simulink model "h2aps_version_final"  (R2024b)
settings: Solver=VariableStepAuto  StartTime=0.0  StopTime=10  RelTol=1e-3
InitFcn:
  | Ts = 1000e-6;
StartFcn:
  | Ts = 1000e-6;
undefined symbols (not defined in the file or in its folder): Ion, Lithium
libraries: slpidlib x13, spsCurrentMeasurementLib x13, simulink x11, spsVoltageMeasurementLib x10, spsSeriesRLCBranchLib x8, spsIGBTDiodeLib x5, spspowerguiLib x2, spsDiodeLib x2, spsBatteryLib x1, spsDCVoltageSourceLib x1, spsVariableResistorLib x1, spsIGBTLib x1
(part 2 of 2)

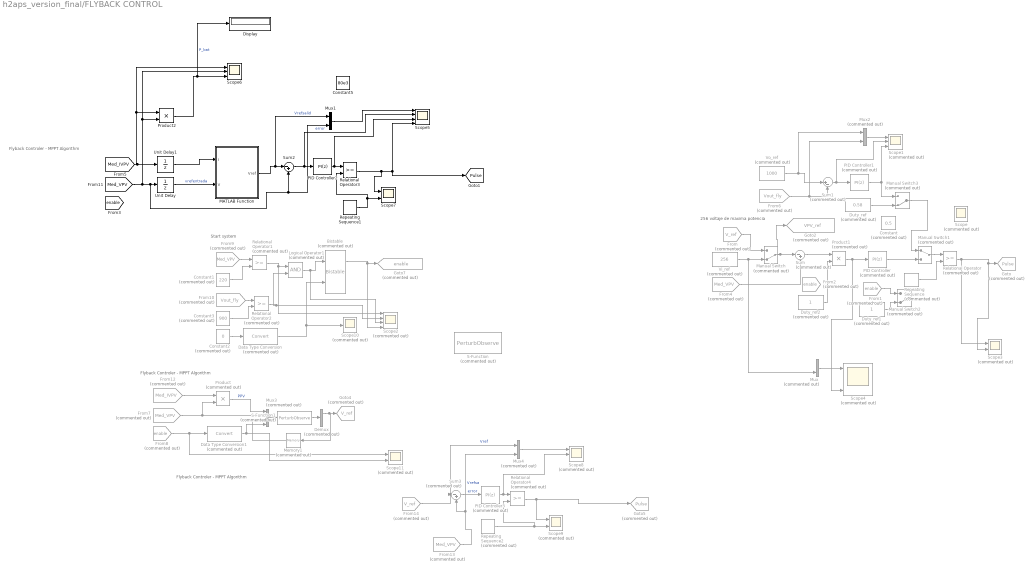
== system h2aps_version_final/FLYBACK CONTROL ==
  note: 256 voltaje de maxima potencia
  note: Flyback Controler - MPPT Algorithm
  note: Start system
  note: Flyback Controler - MPPT Algorithm
  note: Flyback Controler - MPPT Algorithm
  Bistable : spsBistableLib/Bistable  Commented=on  Qpriority=Set  ic=0  Ts=0
      settings: LibrarySourceBlock=sps_lib/Control/Bistable
  Constant : Constant  Commented=on  Value=0.5
  Constant1 : Constant  Commented=on  Value=220
  Constant2 : Constant  Commented=on  Value=0
  Constant3 : Constant  Commented=on  Value=900
  Constant5 : Constant  Value=80e3
  Data Type Conversion : DataTypeConversion  Commented=on  SaturateOnIntegerOverflow=off  RndMeth=Floor
  Data Type Conversion1 : DataTypeConversion  Commented=on  SaturateOnIntegerOverflow=off  RndMeth=Floor
  Demux : Demux  Commented=on  Outputs=3
  Display : Display
  Duty_ref : Constant  Commented=on  Value=0.58
  Duty_ref1 : Constant  Commented=on
  Duty_ref2 : Constant  Commented=on
  From : From  Commented=on  GotoTag=V_ref
  From1 : From  Commented=on  GotoTag=enable
  From10 : From  Commented=on  GotoTag=Vout_fly  TagVisibility=global
  From12 : From  Commented=on  GotoTag=Med_IVPV  TagVisibility=global
  From{4,7,9,13} (4 alike) : From  Commented=on  GotoTag=Med_VPV  TagVisibility=global
  From14 : From  Commented=on  GotoTag=V_ref  TagVisibility=global
  From2 : From  Commented=on  GotoTag=enable
  From6 : From  Commented=on  GotoTag=Vout_fly  TagVisibility=global
  From8 : From  Commented=on  GotoTag=enable  TagVisibility=global
  Goto : Goto  Commented=on  GotoTag=Pulse  TagVisibility=global
  Goto2 : Goto  Commented=on  GotoTag=VPV_ref  TagVisibility=global
  Goto4 : Goto  Commented=on  GotoTag=V_ref  TagVisibility=global
  Goto5 : Goto  Commented=on  GotoTag=Pulse  TagVisibility=global
  Goto7 : Goto  Commented=on  GotoTag=enable  TagVisibility=global
  Logical Operator1 : Logic  Commented=on  AllPortsSameDT=off  OutDataTypeStr=boolean
  MATLAB Function : MATLAB Function  TreatAsAtomicUnit=on
  Manual Switch : ManualSwitch  Commented=on  CurrentSetting=0
  Manual Switch1 : ManualSwitch  Commented=on
  Manual Switch2 : ManualSwitch  Commented=on  CurrentSetting=0
  Manual Switch3 : ManualSwitch  Commented=on  CurrentSetting=0
  Memory1 : Memory  Commented=on
  Mux : Mux  Commented=on  Inputs=2
  Mux1 : Mux  Inputs=2
  Mux2 : Mux  Commented=on  Inputs=2
  Mux3 : Mux  Commented=on
  Mux4 : Mux  Commented=on  Inputs=2
  PID Controller : slpidlib/PID Controller  Commented=on  Controller=PI  Form=Parallel  TimeDomain=Discrete-time  UseExternalTs=off  SampleTime=Ts  IntegratorMethod=Forward Euler  FilterMethod=Forward Euler  ControllerParametersSource=internal  P=0.02/3.2  I=0.04/(2.2*100e-3)  UseKiTs=off  D=0  UseExternalDerivativeSource=off  N=100  UseFilter=on  TunerSelectOption=Transfer Function Based (PID Tuner App)  InitialConditionSource=internal  InitialConditionForIntegrator=0  InitialConditionForFilter=0  DifferentiatorICPrevScaledInput=0  ExternalReset=none  TrackingMode=off  Kt=1  LimitOutput=on  SatLimitsSource=internal  UpperSaturationLimit=1  LowerSaturationLimit=0  LinearizeAsGain=on  AntiWindupMode=clamping  Kb=1  LimitIntegrator=off  UpperIntegratorSaturationLimit=inf  LowerIntegratorSaturationLimit=-inf  POutMin=[]  POutMax=[]  IOutMin=[]  IOutMax=[]  DOutMin=[]  DOutMax=[]  NOutMin=[]  NOutMax=[]  SumOutMin=[]  SumOutMax=[]  SaturationOutMin=[]  SaturationOutMax=[]  PParamMin=[]  PParamMax=[]  IParamMin=[]  IParamMax=[]  DParamMin=[]  DParamMax=[]  NParamMin=[]  NParamMax=[]  KbParamMin=[]  KbParamMax=[]  KtParamMin=[]  KtParamMax=[]  KbOutMin=[]  KbOutMax=[]  KtOutMin=[]  KtOutMax=[]  IntegratorOutMin=[]  IntegratorOutMax=[]  FilterOutMin=[]  FilterOutMax=[]  SumI1OutMin=[]  SumI1OutMax=[]  SumI2OutMin=[]  SumI2OutMax=[]  SumI3OutMin=[]  SumI3OutMax=[]  SumI4OutMin=[]  SumI4OutMax=[]  SumDOutMin=[]  SumDOutMax=[]  DifferentiatorOutMin=[]  DifferentiatorOutMax=[]  FilterDiffOutCoefMin=[]  FilterDiffOutCoefMax=[]  ReciprocalOutMin=[]  ReciprocalOutMax=[]  SumDenOutMin=[]  SumDenOutMax=[]  SumNumOutMin=[]  SumNumOutMax=[]  DivideOutMin=[]  DivideOutMax=[]  UdiffTsProdOutMin=[]  UdiffTsProdOutMax=[]  NTsProdOutMin=[]  NTsProdOutMax=[]  UintegralTsProdOutMin=[]  UintegralTsProdOutMax=[]  UngainTsProdOutMin=[]  UngainTsProdOutMax=[]  ClampingZeroOutDataTypeStr=Inherit: Inherit via back propagation  ClampingZeroOutMin=[]  ClampingZeroOutMax=[]  FilterDenConstantOutDataTypeStr=Inherit: Inherit via back propagation  FilterDenConstantOutMin=[]  FilterDenConstantOutMax=[]  PCopyOutDataTypeStr=Inherit: Inherit via back propagation  PCopyOutMin=[]  PCopyOutMax=[]  NCopyOutDataTypeStr=Inherit: Inherit via back propagation  NCopyOutMin=[]  NCopyOutMax=[]  IntegratorContinuousStateAttributes=''  IntegratorStateMustResolveToSignalObject=off  IntegratorRTWStateStorageClass=Auto  FilterContinuousStateAttributes=''  FilterStateMustResolveToSignalObject=off  FilterRTWStateStorageClass=Auto  ParallelPVariant=InternalParameters  IdealPVariant=Disabled  IVariant=InternalParameters  DVariant=Disabled  IntegratorVariant=Discrete  SatVariant=Enabled  AWVariant=DiscClampingParallel  PCopyVariant=Disabled  TRVariant=Disabled  FdbkBlocksVariant=Forward  IdealPFdbkVariant=Disabled  SatFdbkVariant=Disabled  DerivativeFilterVariant=Disabled  NVariant=Disabled  NCopyVariant=Disabled_SignalSpec  FilterICVariant=Disabled  IntegratorICVariant=InternalICs  ExternalResetVariant=Disabled  TRSumVariant=Passthrough  SumFdbkVariant=Disabled  SumVariant=Sum_PI  TsampFilterVariant=InternalTs  TsampNgainVariant=Passthrough  TsampIntegralVariant=Disabled_SignalSpec  ExternalSaturationOutDataTypeStr=Inherit: Same as second input  DerivativeSourceVariant=Disabled  PreIntVariant=InternalPreInt
  PID Controller1 : slpidlib/PID Controller  Commented=on  Controller=PI  Form=Parallel  TimeDomain=Discrete-time  UseExternalTs=off  SampleTime=Ts  IntegratorMethod=Forward Euler  FilterMethod=Forward Euler  ControllerParametersSource=internal  P=0.02/3.2  I=0.04/(2.2*100e-3)  UseKiTs=off  D=0  UseExternalDerivativeSource=off  N=100  UseFilter=on  TunerSelectOption=Transfer Function Based (PID Tuner App)  InitialConditionSource=internal  InitialConditionForIntegrator=0  InitialConditionForFilter=0  DifferentiatorICPrevScaledInput=0  ExternalReset=none  TrackingMode=off  Kt=1  LimitOutput=on  SatLimitsSource=internal  UpperSaturationLimit=1  LowerSaturationLimit=0  LinearizeAsGain=on  AntiWindupMode=clamping  Kb=1  LimitIntegrator=off  UpperIntegratorSaturationLimit=inf  LowerIntegratorSaturationLimit=-inf  POutMin=[]  POutMax=[]  IOutMin=[]  IOutMax=[]  DOutMin=[]  DOutMax=[]  NOutMin=[]  NOutMax=[]  SumOutMin=[]  SumOutMax=[]  SaturationOutMin=[]  SaturationOutMax=[]  PParamMin=[]  PParamMax=[]  IParamMin=[]  IParamMax=[]  DParamMin=[]  DParamMax=[]  NParamMin=[]  NParamMax=[]  KbParamMin=[]  KbParamMax=[]  KtParamMin=[]  KtParamMax=[]  KbOutMin=[]  KbOutMax=[]  KtOutMin=[]  KtOutMax=[]  IntegratorOutMin=[]  IntegratorOutMax=[]  FilterOutMin=[]  FilterOutMax=[]  SumI1OutMin=[]  SumI1OutMax=[]  SumI2OutMin=[]  SumI2OutMax=[]  SumI3OutMin=[]  SumI3OutMax=[]  SumI4OutMin=[]  SumI4OutMax=[]  SumDOutMin=[]  SumDOutMax=[]  DifferentiatorOutMin=[]  DifferentiatorOutMax=[]  FilterDiffOutCoefMin=[]  FilterDiffOutCoefMax=[]  ReciprocalOutMin=[]  ReciprocalOutMax=[]  SumDenOutMin=[]  SumDenOutMax=[]  SumNumOutMin=[]  SumNumOutMax=[]  DivideOutMin=[]  DivideOutMax=[]  UdiffTsProdOutMin=[]  UdiffTsProdOutMax=[]  NTsProdOutMin=[]  NTsProdOutMax=[]  UintegralTsProdOutMin=[]  UintegralTsProdOutMax=[]  UngainTsProdOutMin=[]  UngainTsProdOutMax=[]  ClampingZeroOutDataTypeStr=Inherit: Inherit via back propagation  ClampingZeroOutMin=[]  ClampingZeroOutMax=[]  FilterDenConstantOutDataTypeStr=Inherit: Inherit via back propagation  FilterDenConstantOutMin=[]  FilterDenConstantOutMax=[]  PCopyOutDataTypeStr=Inherit: Inherit via back propagation  PCopyOutMin=[]  PCopyOutMax=[]  NCopyOutDataTypeStr=Inherit: Inherit via back propagation  NCopyOutMin=[]  NCopyOutMax=[]  IntegratorContinuousStateAttributes=''  IntegratorStateMustResolveToSignalObject=off  IntegratorRTWStateStorageClass=Auto  FilterContinuousStateAttributes=''  FilterStateMustResolveToSignalObject=off  FilterRTWStateStorageClass=Auto  ParallelPVariant=InternalParameters  IdealPVariant=Disabled  IVariant=InternalParameters  DVariant=Disabled  IntegratorVariant=Discrete  SatVariant=Enabled  AWVariant=DiscClampingParallel  PCopyVariant=Disabled  TRVariant=Disabled  FdbkBlocksVariant=Forward  IdealPFdbkVariant=Disabled  SatFdbkVariant=Disabled  DerivativeFilterVariant=Disabled  NVariant=Disabled  NCopyVariant=Disabled_SignalSpec  FilterICVariant=Disabled  IntegratorICVariant=InternalICs  ExternalResetVariant=Disabled  TRSumVariant=Passthrough  SumFdbkVariant=Disabled  SumVariant=Sum_PI  TsampFilterVariant=InternalTs  TsampNgainVariant=Passthrough  TsampIntegralVariant=Disabled_SignalSpec  ExternalSaturationOutDataTypeStr=Inherit: Same as second input  DerivativeSourceVariant=Disabled  PreIntVariant=InternalPreInt
  PID Controller2 : slpidlib/PID Controller  Controller=PI  Form=Parallel  TimeDomain=Discrete-time  UseExternalTs=off  SampleTime=Ts  IntegratorMethod=Forward Euler  FilterMethod=Forward Euler  ControllerParametersSource=internal  P=0.04/3.2  I=0.04/(2.2*100e-3)  UseKiTs=off  D=0  UseExternalDerivativeSource=off  N=100  UseFilter=on  TunerSelectOption=Transfer Function Based (PID Tuner App)  InitialConditionSource=internal  InitialConditionForIntegrator=0  InitialConditionForFilter=0  DifferentiatorICPrevScaledInput=0  ExternalReset=none  TrackingMode=off  Kt=1  LimitOutput=on  SatLimitsSource=internal  UpperSaturationLimit=1  LowerSaturationLimit=0  LinearizeAsGain=on  AntiWindupMode=clamping  Kb=1  LimitIntegrator=off  UpperIntegratorSaturationLimit=inf  LowerIntegratorSaturationLimit=-inf  POutMin=[]  POutMax=[]  IOutMin=[]  IOutMax=[]  DOutMin=[]  DOutMax=[]  NOutMin=[]  NOutMax=[]  SumOutMin=[]  SumOutMax=[]  SaturationOutMin=[]  SaturationOutMax=[]  PParamMin=[]  PParamMax=[]  IParamMin=[]  IParamMax=[]  DParamMin=[]  DParamMax=[]  NParamMin=[]  NParamMax=[]  KbParamMin=[]  KbParamMax=[]  KtParamMin=[]  KtParamMax=[]  KbOutMin=[]  KbOutMax=[]  KtOutMin=[]  KtOutMax=[]  IntegratorOutMin=[]  IntegratorOutMax=[]  FilterOutMin=[]  FilterOutMax=[]  SumI1OutMin=[]  SumI1OutMax=[]  SumI2OutMin=[]  SumI2OutMax=[]  SumI3OutMin=[]  SumI3OutMax=[]  SumI4OutMin=[]  SumI4OutMax=[]  SumDOutMin=[]  SumDOutMax=[]  DifferentiatorOutMin=[]  DifferentiatorOutMax=[]  FilterDiffOutCoefMin=[]  FilterDiffOutCoefMax=[]  ReciprocalOutMin=[]  ReciprocalOutMax=[]  SumDenOutMin=[]  SumDenOutMax=[]  SumNumOutMin=[]  SumNumOutMax=[]  DivideOutMin=[]  DivideOutMax=[]  UdiffTsProdOutMin=[]  UdiffTsProdOutMax=[]  NTsProdOutMin=[]  NTsProdOutMax=[]  UintegralTsProdOutMin=[]  UintegralTsProdOutMax=[]  UngainTsProdOutMin=[]  UngainTsProdOutMax=[]  ClampingZeroOutDataTypeStr=Inherit: Inherit via back propagation  ClampingZeroOutMin=[]  ClampingZeroOutMax=[]  FilterDenConstantOutDataTypeStr=Inherit: Inherit via back propagation  FilterDenConstantOutMin=[]  FilterDenConstantOutMax=[]  PCopyOutDataTypeStr=Inherit: Inherit via back propagation  PCopyOutMin=[]  PCopyOutMax=[]  NCopyOutDataTypeStr=Inherit: Inherit via back propagation  NCopyOutMin=[]  NCopyOutMax=[]  IntegratorContinuousStateAttributes=''  IntegratorStateMustResolveToSignalObject=off  IntegratorRTWStateStorageClass=Auto  FilterContinuousStateAttributes=''  FilterStateMustResolveToSignalObject=off  FilterRTWStateStorageClass=Auto  ParallelPVariant=InternalParameters  IdealPVariant=Disabled  IVariant=InternalParameters  DVariant=Disabled  IntegratorVariant=Discrete  SatVariant=Enabled  AWVariant=DiscClampingParallel  PCopyVariant=Disabled  TRVariant=Disabled  FdbkBlocksVariant=Forward  IdealPFdbkVariant=Disabled  SatFdbkVariant=Disabled  DerivativeFilterVariant=Disabled  NVariant=Disabled  NCopyVariant=Disabled_SignalSpec  FilterICVariant=Disabled  IntegratorICVariant=InternalICs  ExternalResetVariant=Disabled  TRSumVariant=Passthrough  SumFdbkVariant=Disabled  SumVariant=Sum_PI  TsampFilterVariant=InternalTs  TsampNgainVariant=Passthrough  TsampIntegralVariant=Disabled_SignalSpec  ExternalSaturationOutDataTypeStr=Inherit: Same as second input  DerivativeSourceVariant=Disabled  PreIntVariant=InternalPreInt
  PID Controller3 : slpidlib/PID Controller  Commented=on  Controller=PI  Form=Parallel  TimeDomain=Discrete-time  UseExternalTs=off  SampleTime=Ts  IntegratorMethod=Forward Euler  FilterMethod=Forward Euler  ControllerParametersSource=internal  P=0.0062  I=2.8746  UseKiTs=off  D=0  UseExternalDerivativeSource=off  N=100  UseFilter=on  TunerSelectOption=Transfer Function Based (PID Tuner App)  InitialConditionSource=internal  InitialConditionForIntegrator=0  InitialConditionForFilter=0  DifferentiatorICPrevScaledInput=0  ExternalReset=none  TrackingMode=off  Kt=1  LimitOutput=on  SatLimitsSource=internal  UpperSaturationLimit=1  LowerSaturationLimit=0  LinearizeAsGain=on  AntiWindupMode=clamping  Kb=1  LimitIntegrator=off  UpperIntegratorSaturationLimit=inf  LowerIntegratorSaturationLimit=-inf  POutMin=[]  POutMax=[]  IOutMin=[]  IOutMax=[]  DOutMin=[]  DOutMax=[]  NOutMin=[]  NOutMax=[]  SumOutMin=[]  SumOutMax=[]  SaturationOutMin=[]  SaturationOutMax=[]  PParamMin=[]  PParamMax=[]  IParamMin=[]  IParamMax=[]  DParamMin=[]  DParamMax=[]  NParamMin=[]  NParamMax=[]  KbParamMin=[]  KbParamMax=[]  KtParamMin=[]  KtParamMax=[]  KbOutMin=[]  KbOutMax=[]  KtOutMin=[]  KtOutMax=[]  IntegratorOutMin=[]  IntegratorOutMax=[]  FilterOutMin=[]  FilterOutMax=[]  SumI1OutMin=[]  SumI1OutMax=[]  SumI2OutMin=[]  SumI2OutMax=[]  SumI3OutMin=[]  SumI3OutMax=[]  SumI4OutMin=[]  SumI4OutMax=[]  SumDOutMin=[]  SumDOutMax=[]  DifferentiatorOutMin=[]  DifferentiatorOutMax=[]  FilterDiffOutCoefMin=[]  FilterDiffOutCoefMax=[]  ReciprocalOutMin=[]  ReciprocalOutMax=[]  SumDenOutMin=[]  SumDenOutMax=[]  SumNumOutMin=[]  SumNumOutMax=[]  DivideOutMin=[]  DivideOutMax=[]  UdiffTsProdOutMin=[]  UdiffTsProdOutMax=[]  NTsProdOutMin=[]  NTsProdOutMax=[]  UintegralTsProdOutMin=[]  UintegralTsProdOutMax=[]  UngainTsProdOutMin=[]  UngainTsProdOutMax=[]  ClampingZeroOutDataTypeStr=Inherit: Inherit via back propagation  ClampingZeroOutMin=[]  ClampingZeroOutMax=[]  FilterDenConstantOutDataTypeStr=Inherit: Inherit via back propagation  FilterDenConstantOutMin=[]  FilterDenConstantOutMax=[]  PCopyOutDataTypeStr=Inherit: Inherit via back propagation  PCopyOutMin=[]  PCopyOutMax=[]  NCopyOutDataTypeStr=Inherit: Inherit via back propagation  NCopyOutMin=[]  NCopyOutMax=[]  IntegratorContinuousStateAttributes=''  IntegratorStateMustResolveToSignalObject=off  IntegratorRTWStateStorageClass=Auto  FilterContinuousStateAttributes=''  FilterStateMustResolveToSignalObject=off  FilterRTWStateStorageClass=Auto  ParallelPVariant=InternalParameters  IdealPVariant=Disabled  IVariant=InternalParameters  DVariant=Disabled  IntegratorVariant=Discrete  SatVariant=Enabled  AWVariant=DiscClampingParallel  PCopyVariant=Disabled  TRVariant=Disabled  FdbkBlocksVariant=Forward  IdealPFdbkVariant=Disabled  SatFdbkVariant=Disabled  DerivativeFilterVariant=Disabled  NVariant=Disabled  NCopyVariant=Disabled_SignalSpec  FilterICVariant=Disabled  IntegratorICVariant=InternalICs  ExternalResetVariant=Disabled  TRSumVariant=Passthrough  SumFdbkVariant=Disabled  SumVariant=Sum_PI  TsampFilterVariant=InternalTs  TsampNgainVariant=Passthrough  TsampIntegralVariant=Disabled_SignalSpec  ExternalSaturationOutDataTypeStr=Inherit: Same as second input  DerivativeSourceVariant=Disabled  PreIntVariant=InternalPreInt
  Product : Product  Commented=on
  Product1 : Product  Commented=on
  Product2 : Product
  Relational Operator : RelationalOperator  Commented=on  OutDataTypeStr=boolean  InputSameDT=off
  Relational Operator1 : RelationalOperator  Commented=on  OutDataTypeStr=boolean  RndMeth=Simplest  InputSameDT=off
  Relational Operator2 : RelationalOperator  Commented=on  OutDataTypeStr=boolean  RndMeth=Simplest  InputSameDT=off
  Relational Operator3 : RelationalOperator  OutDataTypeStr=boolean  InputSameDT=off
  Relational Operator4 : RelationalOperator  Commented=on  OutDataTypeStr=boolean  InputSameDT=off
  Repeating Sequence : simulink/Sources/Repeating Sequence  Commented=on  rep_seq_t=[0 Ts/2 Ts]  rep_seq_y=[0 1 0]
  Repeating Sequence1 : simulink/Sources/Repeating Sequence  rep_seq_t=[0 Ts/2 Ts]  rep_seq_y=[0 1 0]
  Repeating Sequence2 : simulink/Sources/Repeating Sequence  Commented=on  rep_seq_t=[0 Ts/2 Ts]  rep_seq_y=[0 1 0]
  S-Function : S-Function  Commented=on  FunctionName=PerturbObserve  SFunctionDeploymentMode=off  EnableBusSupport=off
  S-Function1 : S-Function  Commented=on  FunctionName=PerturbObserve  SFunctionDeploymentMode=off  EnableBusSupport=off
  Scope : Scope  Commented=on
  Scope1 : Scope  Commented=on  NumInputPorts=3
  Scope10 : Scope  Commented=on
  Scope11 : Scope  Commented=on  NumInputPorts=2
  Scope2 : Scope  Commented=on  NumInputPorts=4
  Scope3 : Scope  Commented=on  NumInputPorts=2
  Scope4 : Scope  Commented=on  NumInputPorts=3
  Scope5 : Scope  NumInputPorts=4
  Scope6 : Scope  NumInputPorts=3
  Scope7 : Scope  NumInputPorts=2
  Scope8 : Scope  Commented=on  NumInputPorts=3
  Scope9 : Scope  Commented=on  NumInputPorts=2
  Sum : Sum  Commented=on  Inputs=|-+
  Sum1 : Sum  Commented=on  Inputs=|+-
  Sum2 : Sum  Inputs=|-+
  Sum3 : Sum  Commented=on  Inputs=|-+
  Unit Delay : UnitDelay  SampleTime=1e-4  HasFrameUpgradeWarning=on
  Unit Delay1 : UnitDelay  SampleTime=1e-4  HasFrameUpgradeWarning=on
  Vi_ref : Constant  Commented=on  Value=256
  Vo_ref : Constant  Commented=on  Value=1000
  tag scope: Pulse=global
  wires:
  From10/1 -> Relational Operator2/1
  Logical Operator1/1 -> Scope2/3, Bistable/1
  Relational Operator/1 -> Scope3/2, Goto/1, Scope3/1
  Repeating Sequence/1 -> Relational Operator/2
  Constant3/1 -> Relational Operator2/2
  Manual Switch/1 -> Sum/1, Goto2/1
  From9/1 -> Relational Operator1/1
  Constant2/1 -> Data Type Conversion/1
  Constant1/1 -> Relational Operator1/2
  Data Type Conversion/1 -> Bistable/2, Scope10/1
  Sum/1 -> Product1/1
  From/1 -> Manual Switch/1
  From1/1 -> Manual Switch2/1
  Duty_ref1/1 -> Manual Switch2/2
  Duty_ref/1 -> Manual Switch3/2
  Manual Switch3/1 -> Manual Switch1/1
  Sum1/1 -> PID Controller1/1, Scope1/2
  Vo_ref/1 -> Mux2/1, Sum1/1
  From6/1 -> Sum1/2, Mux2/2
  Duty_ref2/1 -> Product1/2
  Vi_ref/1 -> Mux/2, Manual Switch/2
  Mux/1 -> Scope4/1
  Product1/1 -> PID Controller/1, Scope4/3
  Mux2/1 -> Scope1/1
  PID Controller/1 -> Manual Switch1/2
  From4/1 -> Sum/2
  PID Controller1/1 -> Scope1/3, Manual Switch3/1
  Unit Delay1/1 -> MATLAB Function/1(I)
  Sum2/1 -> PID Controller2/1, Scope5/2  "error"
  Unit Delay/1 -> MATLAB Function/2(V)  "vrefentrada"
  Product2/1 -> Display/1, Scope6/3  "P_bat"
  [Med_IVPV] -> Unit Delay1/1, Scope6/1, Product2/1
  [Med_VPV] -> Mux1/2, Sum2/2, Unit Delay/1, Product2/2, Scope6/2
  Mux1/1 -> Scope5/1
  From7/1 -> Product/2, Mux3/2
  From12/1 -> Product/1
  S-Function1/1 -> Demux/1
  Data Type Conversion1/1 -> Scope11/2, Mux3/4
  Mux3/1 -> S-Function1/1
  Memory1/1 -> Mux3/3
  Product/1 -> Mux3/1  "PPV"
  Demux/1 -> Memory1/1, Goto4/1
  Relational Operator4/1 -> Scope9/1, Goto5/1
  Sum3/1 -> PID Controller3/1  "error"
  From14/1 -> Mux4/1, Sum3/1  "Vref"
  PID Controller3/1 -> Scope8/2, Relational Operator4/1
  Mux4/1 -> Scope8/1
  Repeating Sequence2/1 -> Scope9/2, Relational Operator4/2
  From13/1 -> Mux4/2, Sum3/2  "Vrefsa"
  Relational Operator1/1 -> Logical Operator1/1, Scope2/1
  Relational Operator2/1 -> Scope2/2, Logical Operator1/2
  Bistable/1 -> Goto7/1, Scope2/4
  Manual Switch1/1 -> Relational Operator/1
  From8/1 -> Scope11/1, Data Type Conversion1/1
  Relational Operator3/1 -> Scope7/1, Scope5/4, [Pulse]
  Repeating Sequence1/1 -> Scope7/2, Relational Operator3/2
  PID Controller2/1 -> Scope5/3, Relational Operator3/1
  MATLAB Function/1(Vref) -> Mux1/1, Sum2/1  "Vrefsalid"

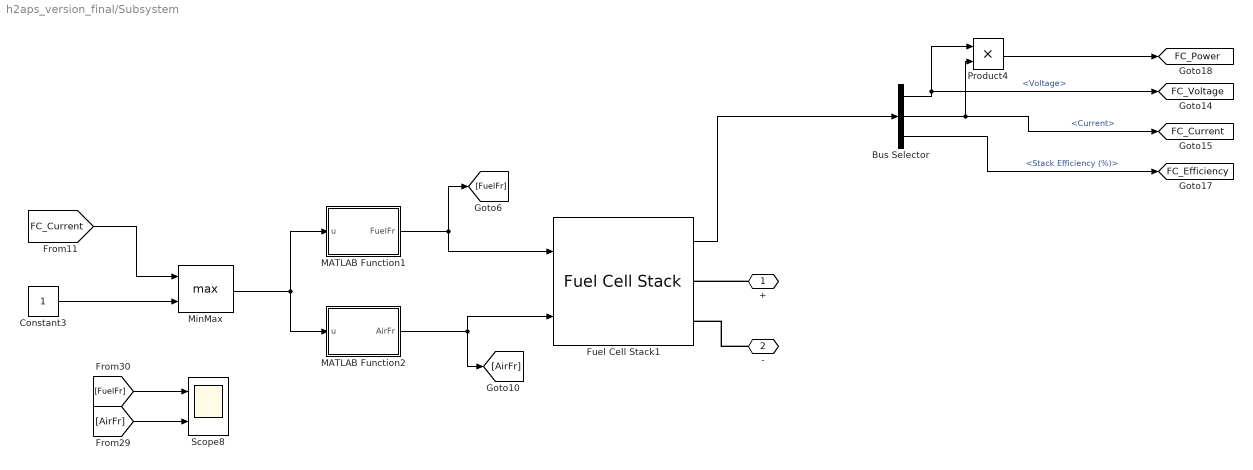
== system h2aps_version_final/Subsystem ==
  Bus Selector : BusSelector  OutputSignals=Voltage,Current,Stack Efficiency (%)
  Constant3 : Constant
  Fuel Cell Stack1 : spsFuelCellStackLib/Fuel Cell Stack  PresetModel=No (User-Defined)  FcType=0  Detailed=Detailed  Eoc=[65,63]  NomVI=[133.3,45]  EndVI=[225,37]  Nc=65  n=55  TOp=65  AirFr=300  SuppPress=[1.5,1]  Comp=[99.95,21,1]  SignX=off  SignY=off  FlowRateH2=on  FlowRateAir=on  SystemTemp=off  SystemPH2=off  SystemPAir=off  FCDyn=off  FC_tau=1  Peak_O2=80  V_Under=10
      settings: LibrarySourceBlock=electricdrivelib/Extra Sources/Fuel Cell Stack
  MATLAB Function1 : MATLAB Function  TreatAsAtomicUnit=on
  MATLAB Function2 : MATLAB Function  TreatAsAtomicUnit=on
  MinMax : MinMax  Function=max  Inputs=2
  Product4 : Product
  Scope8 : Scope  NumInputPorts=2
  + : PMIOPort  Side=Right
  - : PMIOPort  Port=2  Side=Right
  tag scope: FC_Current=global, FC_Efficiency=global, FC_Power=global, FC_Voltage=global
  wires:
  Fuel Cell Stack1/1 -> Bus Selector/1
  MATLAB Function1/1(FuelFr) -> Fuel Cell Stack1/1, [FuelFr]
  MATLAB Function2/1(AirFr) -> Fuel Cell Stack1/2, [AirFr]
  Bus Selector/2 -> Product4/2, [FC_Current]  "<Current>"
  Bus Selector/1 -> Product4/1, [FC_Voltage]  "<Voltage>"
  Product4/1 -> [FC_Power]
  [AirFr] -> Scope8/2
  [FC_Current] -> MinMax/1
  [FuelFr] -> Scope8/1
  Constant3/1 -> MinMax/2
  MinMax/1 -> MATLAB Function1/1(u), MATLAB Function2/1(u)
  Bus Selector/3 -> [FC_Efficiency]  "<Stack Efficiency (%)>"
  connections:
  -/RConn1 -- Fuel Cell Stack1/RConn2
  +/RConn1 -- Fuel Cell Stack1/RConn1

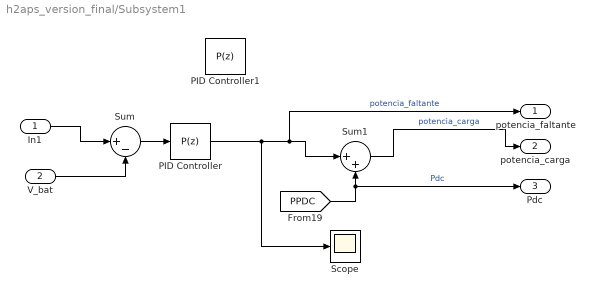
== system h2aps_version_final/Subsystem1 ==
  In1 : Inport
  V_bat : Inport  Port=2
  PID Controller : slpidlib/PID Controller  Controller=P  Form=Parallel  TimeDomain=Discrete-time  UseExternalTs=off  SampleTime=Ts  IntegratorMethod=Forward Euler  FilterMethod=Forward Euler  ControllerParametersSource=internal  P=120  I=50  UseKiTs=off  D=100  UseExternalDerivativeSource=off  N=100  UseFilter=on  TunerSelectOption=Transfer Function Based (PID Tuner App)  InitialConditionSource=internal  InitialConditionForIntegrator=0  InitialConditionForFilter=0  DifferentiatorICPrevScaledInput=0  ExternalReset=none  TrackingMode=off  Kt=1  LimitOutput=on  SatLimitsSource=internal  UpperSaturationLimit=inf  LowerSaturationLimit=-50e3  LinearizeAsGain=on  AntiWindupMode=clamping  Kb=1  LimitIntegrator=off  UpperIntegratorSaturationLimit=inf  LowerIntegratorSaturationLimit=-inf  POutMin=[]  POutMax=[]  IOutMin=[]  IOutMax=[]  DOutMin=[]  DOutMax=[]  NOutMin=[]  NOutMax=[]  SumOutMin=[]  SumOutMax=[]  SaturationOutMin=[]  SaturationOutMax=[]  PParamMin=[]  PParamMax=[]  IParamMin=[]  IParamMax=[]  DParamMin=[]  DParamMax=[]  NParamMin=[]  NParamMax=[]  KbParamMin=[]  KbParamMax=[]  KtParamMin=[]  KtParamMax=[]  KbOutMin=[]  KbOutMax=[]  KtOutMin=[]  KtOutMax=[]  IntegratorOutMin=[]  IntegratorOutMax=[]  FilterOutMin=[]  FilterOutMax=[]  SumI1OutMin=[]  SumI1OutMax=[]  SumI2OutMin=[]  SumI2OutMax=[]  SumI3OutMin=[]  SumI3OutMax=[]  SumI4OutMin=[]  SumI4OutMax=[]  SumDOutMin=[]  SumDOutMax=[]  DifferentiatorOutMin=[]  DifferentiatorOutMax=[]  FilterDiffOutCoefMin=[]  FilterDiffOutCoefMax=[]  ReciprocalOutMin=[]  ReciprocalOutMax=[]  SumDenOutMin=[]  SumDenOutMax=[]  SumNumOutMin=[]  SumNumOutMax=[]  DivideOutMin=[]  DivideOutMax=[]  UdiffTsProdOutMin=[]  UdiffTsProdOutMax=[]  NTsProdOutMin=[]  NTsProdOutMax=[]  UintegralTsProdOutMin=[]  UintegralTsProdOutMax=[]  UngainTsProdOutMin=[]  UngainTsProdOutMax=[]  ClampingZeroOutDataTypeStr=Inherit: Inherit via back propagation  ClampingZeroOutMin=[]  ClampingZeroOutMax=[]  FilterDenConstantOutDataTypeStr=Inherit: Inherit via back propagation  FilterDenConstantOutMin=[]  FilterDenConstantOutMax=[]  PCopyOutDataTypeStr=Inherit: Inherit via back propagation  PCopyOutMin=[]  PCopyOutMax=[]  NCopyOutDataTypeStr=Inherit: Inherit via back propagation  NCopyOutMin=[]  NCopyOutMax=[]  IntegratorContinuousStateAttributes=''  IntegratorStateMustResolveToSignalObject=off  IntegratorRTWStateStorageClass=Auto  FilterContinuousStateAttributes=''  FilterStateMustResolveToSignalObject=off  FilterRTWStateStorageClass=Auto  ParallelPVariant=InternalParameters  IdealPVariant=Disabled  IVariant=Disabled  DVariant=Disabled  IntegratorVariant=Disabled  SatVariant=Enabled  AWVariant=Disabled  PCopyVariant=Disabled  TRVariant=Disabled  FdbkBlocksVariant=Forward  IdealPFdbkVariant=Disabled  SatFdbkVariant=Disabled  DerivativeFilterVariant=Disabled  NVariant=Disabled  NCopyVariant=Disabled_SignalSpec  FilterICVariant=Disabled  IntegratorICVariant=Disabled  ExternalResetVariant=Disabled  TRSumVariant=Passthrough  SumFdbkVariant=Disabled  SumVariant=Passthrough_P  TsampFilterVariant=InternalTs  TsampNgainVariant=Passthrough  TsampIntegralVariant=Disabled_SignalSpec  ExternalSaturationOutDataTypeStr=Inherit: Same as second input  DerivativeSourceVariant=Disabled  PreIntVariant=InternalPreInt
  PID Controller1 : slpidlib/PID Controller  Controller=P  Form=Parallel  TimeDomain=Discrete-time  UseExternalTs=off  SampleTime=Ts  IntegratorMethod=Forward Euler  FilterMethod=Forward Euler  ControllerParametersSource=internal  P=300  I=50  UseKiTs=off  D=100  UseExternalDerivativeSource=off  N=100  UseFilter=on  TunerSelectOption=Transfer Function Based (PID Tuner App)  InitialConditionSource=internal  InitialConditionForIntegrator=0  InitialConditionForFilter=0  DifferentiatorICPrevScaledInput=0  ExternalReset=none  TrackingMode=off  Kt=1  LimitOutput=on  SatLimitsSource=internal  UpperSaturationLimit=3000  LowerSaturationLimit=-3000  LinearizeAsGain=on  AntiWindupMode=clamping  Kb=1  LimitIntegrator=off  UpperIntegratorSaturationLimit=inf  LowerIntegratorSaturationLimit=-inf  POutMin=[]  POutMax=[]  IOutMin=[]  IOutMax=[]  DOutMin=[]  DOutMax=[]  NOutMin=[]  NOutMax=[]  SumOutMin=[]  SumOutMax=[]  SaturationOutMin=[]  SaturationOutMax=[]  PParamMin=[]  PParamMax=[]  IParamMin=[]  IParamMax=[]  DParamMin=[]  DParamMax=[]  NParamMin=[]  NParamMax=[]  KbParamMin=[]  KbParamMax=[]  KtParamMin=[]  KtParamMax=[]  KbOutMin=[]  KbOutMax=[]  KtOutMin=[]  KtOutMax=[]  IntegratorOutMin=[]  IntegratorOutMax=[]  FilterOutMin=[]  FilterOutMax=[]  SumI1OutMin=[]  SumI1OutMax=[]  SumI2OutMin=[]  SumI2OutMax=[]  SumI3OutMin=[]  SumI3OutMax=[]  SumI4OutMin=[]  SumI4OutMax=[]  SumDOutMin=[]  SumDOutMax=[]  DifferentiatorOutMin=[]  DifferentiatorOutMax=[]  FilterDiffOutCoefMin=[]  FilterDiffOutCoefMax=[]  ReciprocalOutMin=[]  ReciprocalOutMax=[]  SumDenOutMin=[]  SumDenOutMax=[]  SumNumOutMin=[]  SumNumOutMax=[]  DivideOutMin=[]  DivideOutMax=[]  UdiffTsProdOutMin=[]  UdiffTsProdOutMax=[]  NTsProdOutMin=[]  NTsProdOutMax=[]  UintegralTsProdOutMin=[]  UintegralTsProdOutMax=[]  UngainTsProdOutMin=[]  UngainTsProdOutMax=[]  ClampingZeroOutDataTypeStr=Inherit: Inherit via back propagation  ClampingZeroOutMin=[]  ClampingZeroOutMax=[]  FilterDenConstantOutDataTypeStr=Inherit: Inherit via back propagation  FilterDenConstantOutMin=[]  FilterDenConstantOutMax=[]  PCopyOutDataTypeStr=Inherit: Inherit via back propagation  PCopyOutMin=[]  PCopyOutMax=[]  NCopyOutDataTypeStr=Inherit: Inherit via back propagation  NCopyOutMin=[]  NCopyOutMax=[]  IntegratorContinuousStateAttributes=''  IntegratorStateMustResolveToSignalObject=off  IntegratorRTWStateStorageClass=Auto  FilterContinuousStateAttributes=''  FilterStateMustResolveToSignalObject=off  FilterRTWStateStorageClass=Auto  ParallelPVariant=InternalParameters  IdealPVariant=Disabled  IVariant=Disabled  DVariant=Disabled  IntegratorVariant=Disabled  SatVariant=Enabled  AWVariant=Disabled  PCopyVariant=Disabled  TRVariant=Disabled  FdbkBlocksVariant=Forward  IdealPFdbkVariant=Disabled  SatFdbkVariant=Disabled  DerivativeFilterVariant=Disabled  NVariant=Disabled  NCopyVariant=Disabled_SignalSpec  FilterICVariant=Disabled  IntegratorICVariant=Disabled  ExternalResetVariant=Disabled  TRSumVariant=Passthrough  SumFdbkVariant=Disabled  SumVariant=Passthrough_P  TsampFilterVariant=InternalTs  TsampNgainVariant=Passthrough  TsampIntegralVariant=Disabled_SignalSpec  ExternalSaturationOutDataTypeStr=Inherit: Same as second input  DerivativeSourceVariant=Disabled  PreIntVariant=InternalPreInt
  Scope : Scope
  Sum : Sum  Inputs=|+-
  Sum1 : Sum  Inputs=|++
  potencia_faltante : Outport
  potencia_carga : Outport  Port=2
  Pdc : Outport  Port=3
  wires:
  Sum1/1 -> potencia_carga/1  "potencia_carga"
  PID Controller/1 -> Scope/1, potencia_faltante/1, Sum1/1  "potencia_faltante"
  V_bat/1 -> Sum/2
  Sum/1 -> PID Controller/1
  [PPDC] -> Pdc/1, Sum1/2  "Pdc"
  In1/1 -> Sum/1

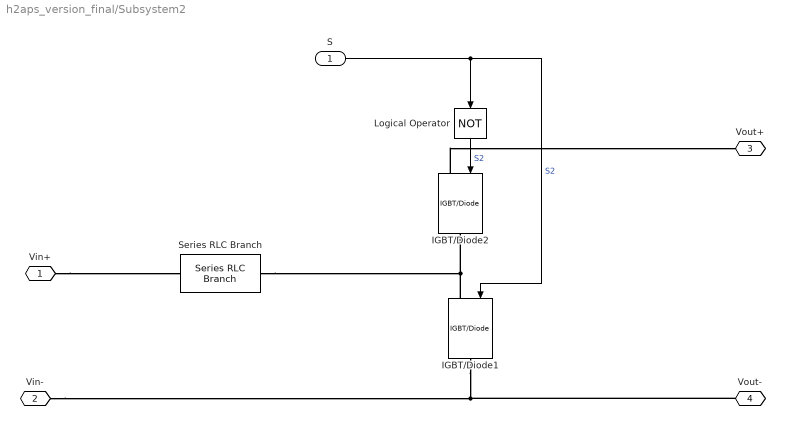
== system h2aps_version_final/Subsystem2 ==
  S : Inport
  IGBT/Diode1 : spsIGBTDiodeLib/IGBT//Diode  Ron=1e-3  Rs=1e5  Cs=inf  Measurements=off
  IGBT/Diode2 : spsIGBTDiodeLib/IGBT//Diode  Ron=1e-3  Rs=1e5  Cs=inf  Measurements=off
  Logical Operator : Logic  Operator=NOT  AllPortsSameDT=off  OutDataTypeStr=boolean
  Series RLC Branch : spsSeriesRLCBranchLib/Series RLC Branch  LConnTagsString=__new0  RConnTagsString=__new0  BranchType=L  Resistance=3  Inductance=100e-3  SetiL0=off  InitialCurrent=0  Capacitance=1e-6  Setx0=off  InitialVoltage=0  Measurements=None
  Vin+ : PMIOPort  Side=Left
  Vin- : PMIOPort  Port=2  Side=Left
  Vout+ : PMIOPort  Port=3  Side=Right
  Vout- : PMIOPort  Port=4  Side=Right
  wires:
  S/1 -> IGBT/Diode1/1, Logical Operator/1  "S2"
  Logical Operator/1 -> IGBT/Diode2/1  "S2"
  connections:
  Vin-/RConn1 -- Vout-/RConn1 -- IGBT/Diode1/RConn1
  Series RLC Branch/RConn1 -- IGBT/Diode1/LConn1 -- IGBT/Diode2/RConn1
  Vin+/RConn1 -- Series RLC Branch/LConn1
  IGBT/Diode2/LConn1 -- Vout+/RConn1

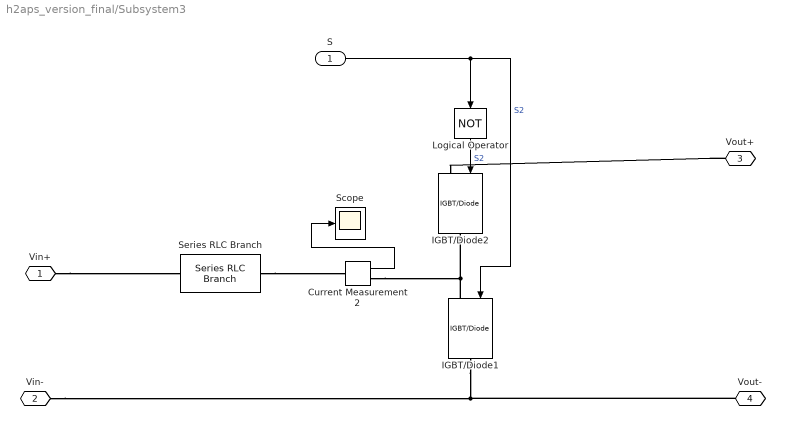
== system h2aps_version_final/Subsystem3 ==
  S : Inport
  Current Measurement2 : spsCurrentMeasurementLib/Current Measurement  PhasorSimulation=off  OutputType=Complex  PSBequivalent=0
  IGBT/Diode1 : spsIGBTDiodeLib/IGBT//Diode  Ron=1e-3  Rs=1e5  Cs=inf  Measurements=off
  IGBT/Diode2 : spsIGBTDiodeLib/IGBT//Diode  Ron=1e-3  Rs=1e5  Cs=inf  Measurements=off
  Logical Operator : Logic  Operator=NOT  AllPortsSameDT=off  OutDataTypeStr=boolean
  Scope : Scope
  Series RLC Branch : spsSeriesRLCBranchLib/Series RLC Branch  LConnTagsString=__new0  RConnTagsString=__new0  BranchType=L  Resistance=3  Inductance=30e-3  SetiL0=off  InitialCurrent=0  Capacitance=1e-6  Setx0=off  InitialVoltage=0  Measurements=None
  Vin+ : PMIOPort  Side=Left
  Vin- : PMIOPort  Port=2  Side=Left
  Vout+ : PMIOPort  Port=3  Side=Right
  Vout- : PMIOPort  Port=4  Side=Right
  wires:
  S/1 -> IGBT/Diode1/1, Logical Operator/1  "S2"
  Logical Operator/1 -> IGBT/Diode2/1  "S2"
  Current Measurement2/1 -> Scope/1
  connections:
  Vin-/RConn1 -- Vout-/RConn1 -- IGBT/Diode1/RConn1
  Series RLC Branch/RConn1 -- Current Measurement2/LConn1
  Vin+/RConn1 -- Series RLC Branch/LConn1
  Vout+/RConn1 -- IGBT/Diode2/LConn1
  IGBT/Diode1/LConn1 -- Current Measurement2/RConn1 -- IGBT/Diode2/RConn1

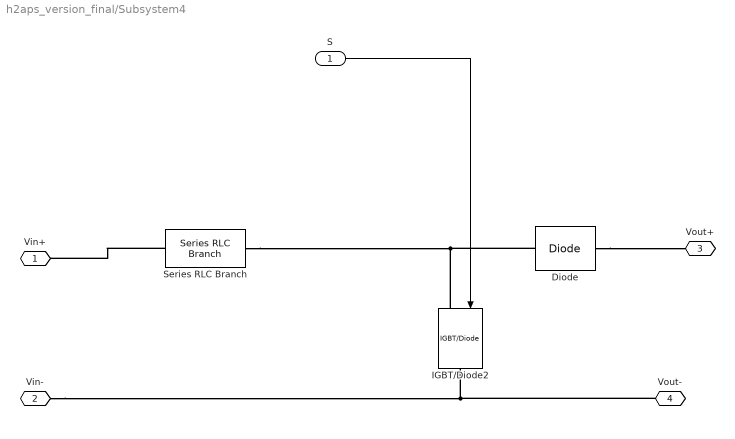
== system h2aps_version_final/Subsystem4 ==
  S : Inport
  Diode : spsDiodeLib/Diode  Ron=0.001  Lon=0  Vf=0.8  IC=0  UseSnubber=0  Rs=500  Cs=250e-9  Measurements=off
  IGBT/Diode2 : spsIGBTDiodeLib/IGBT//Diode  Ron=1e-3  Rs=1e5  Cs=inf  Measurements=off
  Series RLC Branch : spsSeriesRLCBranchLib/Series RLC Branch  LConnTagsString=__new0  RConnTagsString=__new0  BranchType=L  Resistance=3  Inductance=1e-2  SetiL0=off  InitialCurrent=0  Capacitance=1e-6  Setx0=off  InitialVoltage=0  Measurements=None
  Vin+ : PMIOPort  Side=Left
  Vin- : PMIOPort  Port=2  Side=Left
  Vout+ : PMIOPort  Port=3  Side=Right
  Vout- : PMIOPort  Port=4  Side=Right
  wires:
  S/1 -> IGBT/Diode2/1
  connections:
  Vin-/RConn1 -- Vout-/RConn1 -- IGBT/Diode2/RConn1
  Diode/RConn1 -- Vout+/RConn1
  Series RLC Branch/RConn1 -- Vin+/RConn1
  Diode/LConn1 -- Series RLC Branch/LConn1 -- IGBT/Diode2/LConn1

== system h2aps_version_final/Subsystem6 ==
  Supercapacitor : spsSupercapacitorLib/Supercapacitor  C=5.5  Rdc=1.86e-3  Voltage=400  Ns=6  Np=1  Vinit=360  Temp=25  Nc=1  r=1e-9  epsilon=6.0208e-10  Ioc=10  Vself="[48  47.8  47.06  44.65]"
      settings: LibrarySourceBlock=electricdrivelib/Extra Sources/Supercapacitor
  V+ : PMIOPort  Side=Left
  V- : PMIOPort  Port=2  Side=Left
  m : Outport
  wires:
  Supercapacitor/1 -> m/1
  connections:
  Supercapacitor/LConn1 -- V+/RConn1
  Supercapacitor/LConn2 -- V-/RConn1

== matlab function h2aps_version_final/MATLAB Function ==
  data: ECB input; ECU input; PBAT output; PUC output; PC output; PCC input; M input; PCAR input; boolsalida output; boolentrada input; contador2 input
%BLOQUE DE H2APS 
function [PBAT,PUC,PC,boolsalida ]  = P_UCs(ECB,ECU,PCC, M, PCAR,boolentrada,contador2)
% Parámetros de los componentes
capacidad_bateria=70000 ; % Capacidad total de la batería en kWh
capacidad_ultracapacitor =40000; % Capacidad total del ultracapacitor en kWh
%Parametros de entrada de la funcion
potencia_celda_combustible=PCC ; % Potencia de la celda de combustible en kW
potencia_carga=PCAR; % Potencia de la carga  en kW

soc_bateria =ECB; % Cantidad de potencia que tiene la bateria en determinado momento kW
soc_ultracapacitor =ECU; % kWh Cantidad de potencia que tinee el ultracapacitor en determiando momento kw


%condicion inicial
demanda_actual = potencia_carga;
potencia_disponible = potencia_celda_combustible;
persistent dato dato2;

if isempty(dato)
    dato=0;
    dato2=0
end

        
    if demanda_actual <= potencia_disponible
       potencia_distribuida_motor = demanda_actual;
       potencia_extraida=0;
    else
       % Calcular la cantidad de energía que se extraerá de la batería
       potencia_extraida = demanda_actual - potencia_disponible;
       % Restar esta energía extraída de la batería al estado de carga de la batería
       % soc_bateria = max(soc_bateria - potencia_extraida_bateria, 0);
       potencia_distribuida_motor = potencia_disponible+potencia_extraida;
    end
    
    PC=potencia_distribuida_motor;
    % Calcular la energía sobrante después de satisfacer la demanda del motor
    potencia_sobrante =potencia_disponible -potencia_distribuida_motor;
  
         
     % Calcular la proporción de energía a distribuir a la batería y al ultracapacitor
       potencia_distribuida_bateria=potencia_sobrante;       
       PBAT=-(0.8* potencia_distribuida_bateria);  % los valores deben ser negtaivos para que absorba la energia sobrante, pero solo el 80%
       if potencia_sobrante>=-200  
            if (M>=1e4 || M<-1e4) 
                   
                    boolsalida=true;
                    potencia_distribuida_ultracapacitor=5e3;
                    PUC=-potencia_distribuida_ultracapacitor;
                    dato=contador2;
            else
                if boolentrada==1   %que solo absorba hasta que el soc llegue a 0.88   
                   
                    if contador2-dato<0.0039
                        potencia_distribuida_ultracapacitor=5e3;
                        PUC=-potencia_distribuida_ultracapacitor;
                       
                        boolsalida=true;
                    else
                        potencia_distribuida_ultracapacitor=0;
                        PUC=-potencia_distribuida_ultracapacitor;
                        
                        boolsalida=false;
                    end
                 %   PA=0;
                %%%Rrevisar esta distribucion de potencia 
                else                              %si pasa este valor que el capacitor se vaya a cero
                    potencia_distribuida_ultracapacitor=0;
                    PUC=potencia_distribuida_ultracapacitor;
                   
                   
                    boolsalida=false;
                end 
            end 
       else 
            
          potencia_distribuida_bateria=potencia_extraida;        
          PBAT=1.2*potencia_distribuida_bateria;  % los valores deben ser positivos para que de la energia que falta
 
             
                if(M>1e4 || M<-1e4 )
                  potencia_distribuida_ultracapacitor=5e3;
                  PUC=potencia_distribuida_ultracapacitor;
                  dato2=contador2;
                  boolsalida=true;
                else
                    if boolentrada==1   %que solo absorba hasta que el soc llegue a 0.88   

                        if dato2-contador2<0.0039
                            potencia_distribuida_ultracapacitor=5e3;
                            PUC=potencia_distribuida_ultracapacitor;
                            
                            boolsalida=true;
                        else
                            potencia_distribuida_ultracapacitor=0;
                            PUC=potencia_distribuida_ultracapacitor;
                           
                            boolsalida=false;
                        end
                     %   PA=0;
                    %%%Rrevisar esta distribucion de potencia 
                    else                              %si pasa este valor que el capacitor se vaya a cero
                        potencia_distribuida_ultracapacitor=0;
                        PUC=potencia_distribuida_ultracapacitor;

                     
                        boolsalida=false;
                    end 
                end
      end

== matlab function h2aps_version_final/Subsystem/MATLAB Function1 ==
  data: u input; FuelFr output
function FuelFr = fcn(u)
FuelFr=6000*8.3145*(273+95)*400*u(1)/(2*9648*(3*101325)*0.919*0.995);

== matlab function h2aps_version_final/Subsystem/MATLAB Function2 ==
  data: u input; AirFr output
function AirFr = fcn(u)
AirFr=6000*8.3145*(273+95)*400*u(1)/(4*9648*(3*101325)*0.5057*0.21);

== matlab function h2aps_version_final/FLYBACK CONTROL/MATLAB Function ==
  data: I input; Vref output; V input
function Vref = CTR(I,V)

Vrefmax=270;
Vrefinit=256;
Vrefmini=235;
deltaVref=1;
persistent Vold Pold Vrefold;
if isempty(Vold)
    Vold=200;
    Pold=80000;
    Vrefold=Vrefinit;
end
P=V*I;
dV= V-Vold;
dP= P-Pold;

if (dP~=0)
    if dP<0
        if dV<0
             Vref = Vrefold+deltaVref;
        else
             Vref = Vrefold-deltaVref;
        end
        
    else
        if dV<0
            Vref = Vrefold-deltaVref;
        else
            Vref = Vrefold+deltaVref;
        end
    end    
else 
  Vref= Vrefold;
    
end

if Vref >= Vrefmax || Vref <= Vrefmini
    Vref = 260;
    
end
Vrefold = Vref;
Vold=V;
Pold=P;
